simulink model "P7_Cascade_Control"  (R2023b)
settings: Solver=FixedStepAuto  StartTime=0.0  StopTime=20e-3  FixedStep=1e-8  RelTol=1e-3
values from neighbouring files (symbols this model uses):
  L = 2e-3    (= 0.002)    [P7_T1_Buck_Single_Loop.m]
libraries: spsSeriesRLCBranchLib x9, spsMeanLib x6, spsCurrentMeasurementLib x3, spsDiodeLib x3, spsIdealSwitchLib x3, eePwmGenerator x3, spsDCVoltageSourceLib x3, spsVoltageMeasurementLib x3, slpidlib x2, sps_lib x1
settings Model: Creator=Lucas  LastModifiedBy=Lucas
settings SolverCC: ZeroCrossAlgorithm=Adaptive
settings DebuggingCC: IgnoredZcDiagnostic=none

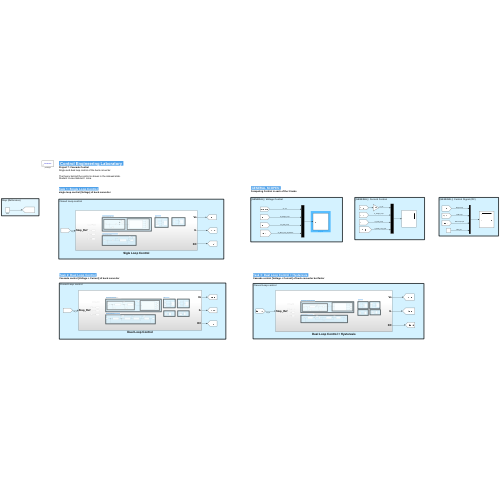
[thumbnail: Simulink's stored preview of the top-level diagram]
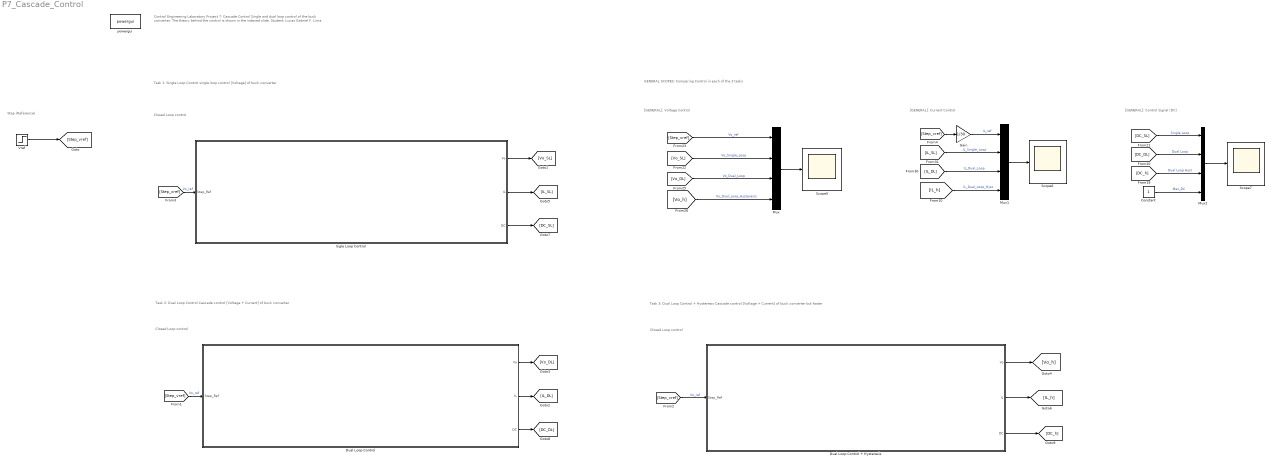
== system P7_Cascade_Control ==
  note: Control Engineering Laboratory
      | Project 7: Cascade Control
      | Single and dual loop control of the buck converter.
      |
      | The theory behind the control is shown in the indexed slide.
      | Student: Lucas Gabriel F. Lima.
  note: Step (Reference)
  note: [GENERAL]: Voltage Control
  note: [GENERAL]: Current Control
  note: [GENERAL]: Control Signal (DC)
  note: GENERAL SCOPES:
      | Comparing Control in each of the 3 tasks
  note: Task 2: Dual Loop Control
      | Cascade control [Voltage + Current] of buck converter
  note: Task 3: Dual Loop Control + Hysteresis
      | Cascade control [Voltage + Current] of buck converter but faster
  note: Task 1: Single Loop Control
      | single loop control [Voltage] of buck converter
  note: Closed Loop control
  note: Closed Loop control
  note: Closed Loop control
  Constant : Constant
  Dual Loop Control : Subsystem
  Dual Loop Control + Hysteresis : Subsystem
  Gain : Gain  Gain=1/30
  Mux : Mux
  Mux1 : Mux
  Mux2 : Mux
  Scope5 : Scope
  Scope6 : Scope
  Scope7 : Scope
  Sigle Loop Control : Subsystem
  Vref : Step  Time=10e-3  Before=60  After=66  SampleTime=0
  powergui : sps_lib/powergui  Priority=1  SimulationMode=Continuous  SampleTime=50e-6  frequency=60  Iterations=50  frequencyindice=0  Pbase=100e6  ErrMax=1e-4  UnitsV=kV  UnitsW=MW  buscounter=0  FunctionMessages=off  echomessages=off  EnableUseOfTLC=off  CurrentSourceSwitches=off  DisableSnubberDevices=off  DisableRonSwitches=off  DisableVfSwitches=off  DisplayEquations=off  AutomaticDiscreteSolvers=off  SolverType=Tustin/Backward Euler (TBE)  Interpol=off  ExternalGateDelay=off  methode=off  Ts=100  x0status=blocks  SPID=on  SwTol=0  HookPort=off  NonlinearTolerance=1e-4  nMaxIteration=100  ContinueOnMaxIteration=off  RestoreLinks=warning  ResistiveCurrentMeasurement=off  Frange=[0:2:500]  Ylog=off  Xlog=on  ShowGrid=off  save=off  variable=ZData  structure=0  ZoomFFT=off  StartTime=0.0  cycles=1  DisplayStyle=1  fundamental=60  FreqAxis=off  MaxFrequency=1000  frequencyindicesteady=1  RmsSteady=1  display=off
  wires:
  Vref/1 -> [Step_vref]
  [DC_h] -> Mux2/3  "Dual Loop Hyst"
  [DC_DL] -> Mux2/2  "Dual Loop"
  [DC_SL] -> Mux2/1  "Single Loop"
  [Vo_SL] -> Mux/2  "Vo_Single_Loop"
  [Step_vref] -> Mux/1  "Vo_ref"
  [Vo_DL] -> Mux/3  "Vo_Dual_Loop"
  [Vo_h] -> Mux/4  "Vo_Dual_Loop_Hysteresis"
  Mux/1 -> Scope5/1
  [IL_h] -> Mux1/4  "IL_Dual_Loop_Hyst"
  [IL_DL] -> Mux1/3  "IL_Dual_Loop"
  [IL_SL] -> Mux1/2  "IL_Single_Loop"
  Mux1/1 -> Scope6/1
  Mux2/1 -> Scope7/1
  Constant/1 -> Mux2/4  "Max_DC"
  [Step_vref] -> Dual Loop Control/1(Step_Ref)  "Vo_ref"
  Dual Loop Control/1(Vo) -> [Vo_DL]
  Dual Loop Control/2(IL) -> [IL_DL]
  [Step_vref] -> Dual Loop Control + Hysteresis/1(Step_Ref)  "Vo_ref"
  Dual Loop Control + Hysteresis/1(Vo) -> [Vo_h]
  Dual Loop Control + Hysteresis/2(IL) -> [IL_h]
  [Step_vref] -> Sigle Loop Control/1(Step_Ref)  "Vo_ref"
  Sigle Loop Control/1(Vo) -> [Vo_SL]
  Sigle Loop Control/2(IL) -> [IL_SL]
  Sigle Loop Control/3(DC) -> [DC_SL]
  Dual Loop Control/3(DC) -> [DC_DL]
  Dual Loop Control + Hysteresis/3(DC) -> [DC_h]
  [Step_vref] -> Gain/1
  Gain/1 -> Mux1/1  "IL_ref"

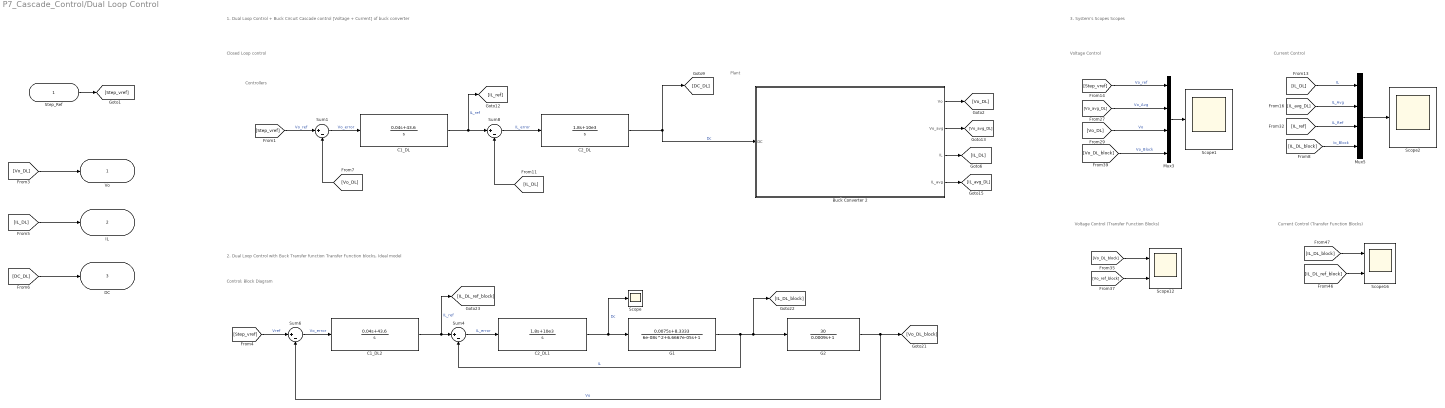
== system P7_Cascade_Control/Dual Loop Control ==
  note: Closed Loop control
  note: Control: Block Diagram
  note: Controllers
  note: Plant
  note: Voltage Control
  note: Current Control
  note: 1. Dual Loop Control + Buck Circuit
      | Cascade control [Voltage + Current] of buck converter
  note: 2. Dual Loop Control with Buck Transfer function
      | Transfer Function blocks, Ideal model
  note: 3. System's Scopes
      | Scopes
  note: Voltage Control (Transfer Function Blocks)
  note: Current Control (Transfer Function Blocks)
  Step_Ref : Inport
  Buck Converter 2 : Subsystem
  C1_DL : TransferFcn  Numerator=[0.04, 43.6]  Denominator=[1 , 0]
  C1_DL2 : TransferFcn  Numerator=[0.04, 43.6]  Denominator=[1 , 0]
  C2_DL : TransferFcn  Numerator=[1.8, 10e3]  Denominator=[1, 0]
  C2_DL1 : TransferFcn  Numerator=[1.8, 10e3]  Denominator=[1, 0]
  G1 : TransferFcn  Numerator=[0.0075, 8.3333]  Denominator=[6e-08, 6.6667e-05 ,1]
  G2 : TransferFcn  Numerator=30  Denominator=[0.0009 1]
  Mux3 : Mux
  Mux5 : Mux
  Scope : Scope
  Scope1 : Scope
  Scope12 : Scope  NumInputPorts=2
  Scope16 : Scope  NumInputPorts=2
  Scope2 : Scope
  Sum{1,4,6,8} (4 alike) : Sum  Inputs=|+-
  Vo : Outport
  IL : Outport  Port=2
  DC : Outport  Port=3
  wires:
  Sum6/1 -> C1_DL2/1  "Vo_error"
  Buck Converter 2/1(Vo) -> [Vo_DL]
  [IL_avg_DL] -> Mux5/2  "IL_Avg"
  [Step_vref] -> Sum6/1  "Vref"
  [Vo_DL] -> Sum1/2
  Sum4/1 -> C2_DL1/1  "IL_error"
  G1/1 -> [IL_DL_block], G2/1, Sum4/2  "IL"
  C1_DL2/1 -> [IL_DL_ref_block], Sum4/1  "IL_ref"
  [IL_DL] -> Mux5/1  "IL"
  [Vo_DL_block] -> Scope12/1
  Mux3/1 -> Scope1/1
  Sum1/1 -> C1_DL/1  "Vo_error"
  [IL_DL] -> Sum8/2
  Sum8/1 -> C2_DL/1  "IL_error"
  Buck Converter 2/3(IL) -> [IL_DL]
  C2_DL/1 -> Buck Converter 2/1(DC), [DC_DL]  "Dc"
  G2/1 -> [Vo_DL_block], Sum6/2  "Vo"
  C2_DL1/1 -> Scope/1, G1/1  "Dc"
  [IL_ref] -> Mux5/3  "IL_Ref"
  [Vo_ref_block] -> Scope12/2
  [Vo_avg_DL] -> Mux3/2  "Vo_Avg"
  Buck Converter 2/4(IL_avg) -> [IL_avg_DL]
  C1_DL/1 -> [IL_ref], Sum8/1  "IL_ref"
  [IL_DL_block] -> Scope16/1
  [Vo_DL] -> Mux3/3  "Vo"
  [Step_vref] -> Sum1/1  "Vo_ref"
  [Step_vref] -> Mux3/1  "Vo_ref"
  [Vo_DL_block] -> Mux3/4  "Vo_Block"
  Buck Converter 2/2(Vo_avg) -> [Vo_avg_DL]
  [IL_DL_block] -> Mux5/4  "Io_Block"
  Mux5/1 -> Scope2/1
  [IL_DL_ref_block] -> Scope16/2
  Step_Ref/1 -> [Step_vref]
  [Vo_DL] -> Vo/1
  [DC_DL] -> DC/1
  [IL_DL] -> IL/1

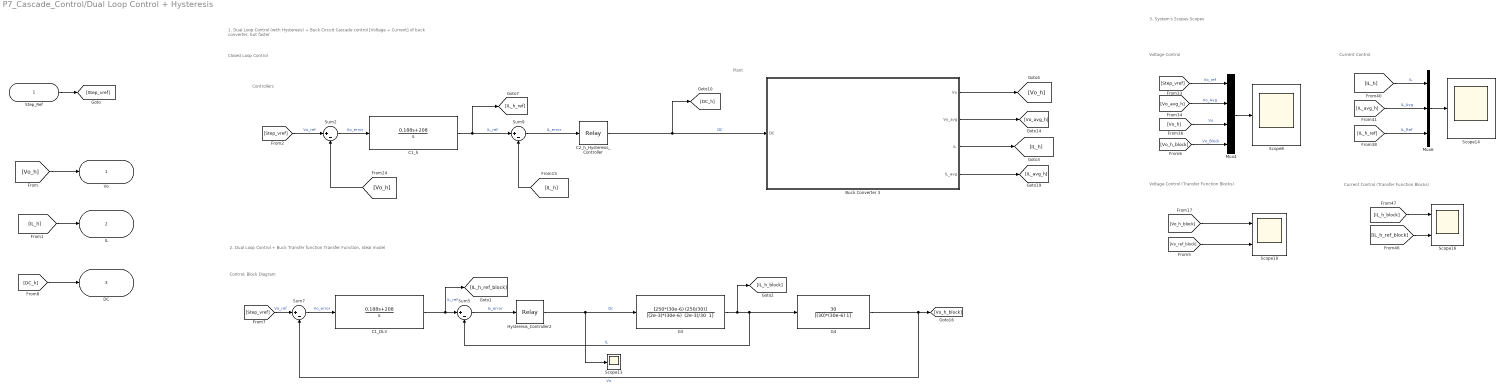
== system P7_Cascade_Control/Dual Loop Control + Hysteresis ==
  note: 2. Dual Loop Control + Buck Transfer function
      | Transfer Function, Ideal model
  note: Control: Block Diagram
  note: Controllers
  note: 1. Dual Loop Control (with Hysteresis) + Buck Circuit
      | Cascade control [Voltage + Current] of buck converter, but faster
  note: Voltage Control
  note: Plant
  note: Current Control
  note: Closed Loop Control
  note: 3. System's Scopes
      | Scopes
  note: Voltage Control (Transfer Function Blocks)
  note: Current Control (Transfer Function Blocks)
  Step_Ref : Inport
  Buck Converter 3 : Subsystem
  C1_DL3 : TransferFcn  Numerator=[0.188 , 208]  Denominator=[1 , 0]
  C1_h : TransferFcn  Numerator=[0.188 , 208]  Denominator=[1 , 0]
  C2_h_Hysteresis_Controller : Relay  OnSwitchValue=0.2/2  OffSwitchValue=-0.2/2
  G3 : TransferFcn  Numerator=[250*(30e-6) (250/30)]  Denominator="[(2e-3)*(30e-6)  (2e-3)/30  1]"
  G4 : TransferFcn  Numerator=30  Denominator=[(30)*(30e-6) 1]
  Hysteresis_Controller2 : Relay  OnSwitchValue=0.2/2  OffSwitchValue=-0.2/2
  Mux4 : Mux
  Mux6 : Mux  Inputs=3
  Scope10 : Scope  NumInputPorts=2
  Scope13 : Scope
  Scope14 : Scope
  Scope16 : Scope  NumInputPorts=2
  Scope8 : Scope
  Sum{2,5,7,9} (4 alike) : Sum  Inputs=|+-
  Vo : Outport
  IL : Outport  Port=2
  DC : Outport  Port=3
  wires:
  G3/1 -> [IL_h_block], G4/1, Sum5/2  "IL"
  Sum7/1 -> C1_DL3/1  "Vo_error"
  C1_DL3/1 -> [IL_h_ref_block], Sum5/1  "IL_ref"
  C1_h/1 -> [IL_h_ref], Sum9/1  "IL_ref"
  G4/1 -> Sum7/2, [Vo_h_block]  "Vo"
  [Vo_ref_block] -> Scope10/2
  [Vo_avg_h] -> Mux4/2  "Vo_Avg"
  [Vo_h_block] -> Scope10/1
  Buck Converter 3/3(IL) -> [IL_h]
  Mux4/1 -> Scope8/1
  Sum5/1 -> Hysteresis_Controller2/1  "Io_error"
  [IL_h] -> Sum9/2
  C2_h_Hysteresis_Controller/1 -> Buck Converter 3/1(DC), [DC_h]  "DC"
  Buck Converter 3/1(Vo) -> [Vo_h]
  [Vo_h] -> Sum2/2
  [Vo_h] -> Mux4/3  "Vo"
  Sum9/1 -> C2_h_Hysteresis_Controller/1  "IL_error"
  [IL_avg_h] -> Mux6/2  "IL_Avg"
  Sum2/1 -> C1_h/1  "Vo_error"
  [IL_h_ref] -> Mux6/3  "IL_Ref"
  Buck Converter 3/4(IL_avg) -> [IL_avg_h]
  Mux6/1 -> Scope14/1
  Buck Converter 3/2(Vo_avg) -> [Vo_avg_h]
  [Step_vref] -> Mux4/1  "Vo_ref"
  Hysteresis_Controller2/1 -> Scope13/1, G3/1  "Dc"
  [Step_vref] -> Sum2/1  "Vo_ref"
  [IL_h] -> Mux6/1  "IL"
  Step_Ref/1 -> [Step_vref]
  [Vo_h] -> Vo/1
  [Vo_h_block] -> Mux4/4  "Vo_Block"
  [Step_vref] -> Sum7/1  "Vo_ref"
  [DC_h] -> DC/1
  [IL_h_ref_block] -> Scope16/2
  [IL_h_block] -> Scope16/1
  [IL_h] -> IL/1

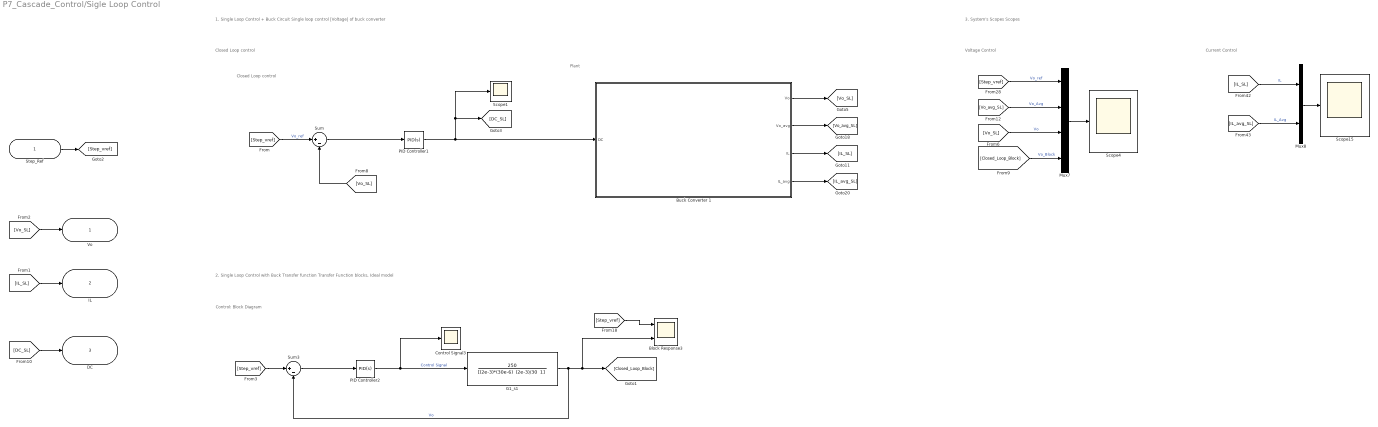
== system P7_Cascade_Control/Sigle Loop Control ==
  note: Closed Loop control
  note: Control: Block Diagram
  note: Voltage Control
  note: Current Control
  note: Plant
  note: Closed Loop control
  note: 1. Single Loop Control + Buck Circuit
      | Single loop control [Voltage] of buck converter
  note: 2. Single Loop Control with Buck Transfer function
      | Transfer Function blocks, Ideal model
  note: 3. System's Scopes
      | Scopes
  Step_Ref : Inport
  Block Response3 : Scope  NumInputPorts=2
  Buck Converter 1 : Subsystem
  Control Signal3 : Scope
  G1_s1 : TransferFcn  Numerator=250  Denominator="[(2e-3)*(30e-6)  (2e-3)/30  1]"
  Mux7 : Mux
  Mux8 : Mux  Inputs=2
  PID Controller1 : slpidlib/PID Controller  Controller=PID  Form=Parallel  TimeDomain=Continuous-time  UseExternalTs=off  SampleTime=-1  IntegratorMethod=Forward Euler  FilterMethod=Forward Euler  ControllerParametersSource=internal  P=0.0075  I=14  UseKiTs=off  D=0.8e-06  N=1/(8.18e-06)  UseFilter=on  TunerSelectOption=Transfer Function Based (PID Tuner App)  InitialConditionSource=internal  InitialConditionForIntegrator=0  InitialConditionForFilter=0  DifferentiatorICPrevScaledInput=0  ExternalReset=none  TrackingMode=off  Kt=1  LimitOutput=off  SatLimitsSource=internal  UpperSaturationLimit=inf  LowerSaturationLimit=-inf  LinearizeAsGain=on  AntiWindupMode=none  Kb=1  LimitIntegrator=off  UpperIntegratorSaturationLimit=inf  LowerIntegratorSaturationLimit=-inf  POutMin=[]  POutMax=[]  IOutMin=[]  IOutMax=[]  DOutMin=[]  DOutMax=[]  NOutMin=[]  NOutMax=[]  SumOutMin=[]  SumOutMax=[]  SaturationOutMin=[]  SaturationOutMax=[]  PParamMin=[]  PParamMax=[]  IParamMin=[]  IParamMax=[]  DParamMin=[]  DParamMax=[]  NParamMin=[]  NParamMax=[]  KbParamMin=[]  KbParamMax=[]  KtParamMin=[]  KtParamMax=[]  KbOutMin=[]  KbOutMax=[]  KtOutMin=[]  KtOutMax=[]  IntegratorOutMin=[]  IntegratorOutMax=[]  FilterOutMin=[]  FilterOutMax=[]  SumI1OutMin=[]  SumI1OutMax=[]  SumI2OutMin=[]  SumI2OutMax=[]  SumI3OutMin=[]  SumI3OutMax=[]  SumI4OutMin=[]  SumI4OutMax=[]  SumDOutMin=[]  SumDOutMax=[]  DifferentiatorOutMin=[]  DifferentiatorOutMax=[]  FilterDiffOutCoefMin=[]  FilterDiffOutCoefMax=[]  ReciprocalOutMin=[]  ReciprocalOutMax=[]  SumDenOutMin=[]  SumDenOutMax=[]  SumNumOutMin=[]  SumNumOutMax=[]  DivideOutMin=[]  DivideOutMax=[]  UdiffTsProdOutMin=[]  UdiffTsProdOutMax=[]  NTsProdOutMin=[]  NTsProdOutMax=[]  UintegralTsProdOutMin=[]  UintegralTsProdOutMax=[]  UngainTsProdOutMin=[]  UngainTsProdOutMax=[]  ClampingZeroOutDataTypeStr=Inherit: Inherit via back propagation  ClampingZeroOutMin=[]  ClampingZeroOutMax=[]  FilterDenConstantOutDataTypeStr=Inherit: Inherit via back propagation  FilterDenConstantOutMin=[]  FilterDenConstantOutMax=[]  PCopyOutDataTypeStr=Inherit: Inherit via back propagation  PCopyOutMin=[]  PCopyOutMax=[]  NCopyOutDataTypeStr=Inherit: Inherit via back propagation  NCopyOutMin=[]  NCopyOutMax=[]  IntegratorContinuousStateAttributes=''  IntegratorStateMustResolveToSignalObject=off  IntegratorRTWStateStorageClass=Auto  FilterContinuousStateAttributes=''  FilterStateMustResolveToSignalObject=off  FilterRTWStateStorageClass=Auto  ParallelPVariant=InternalParameters  IdealPVariant=Disabled  IVariant=InternalParameters  DVariant=InternalParameters  IntegratorVariant=Continuous  SatVariant=Disabled  AWVariant=Passthrough  PCopyVariant=Disabled  TRVariant=Disabled  FdbkBlocksVariant=Forward  IdealPFdbkVariant=Disabled  SatFdbkVariant=Disabled  DerivativeFilterVariant=ContFilter  NVariant=InternalParameters  NCopyVariant=Disabled  FilterICVariant=InternalICsFilter  IntegratorICVariant=InternalICs  ExternalResetVariant=Disabled  TRSumVariant=Passthrough  SumFdbkVariant=Disabled  SumVariant=Sum_PID  TsampFilterVariant=InternalTs  TsampNgainVariant=Passthrough  TsampIntegralVariant=Disabled_SignalSpec  ExternalSaturationOutDataTypeStr=Inherit: Same as second input
  PID Controller2 : slpidlib/PID Controller  Controller=PID  Form=Parallel  TimeDomain=Continuous-time  UseExternalTs=off  SampleTime=-1  IntegratorMethod=Forward Euler  FilterMethod=Forward Euler  ControllerParametersSource=internal  P=0.0075  I=14  UseKiTs=off  D=0.8e-06  N=1/(8.18e-06)  UseFilter=on  TunerSelectOption=Transfer Function Based (PID Tuner App)  InitialConditionSource=internal  InitialConditionForIntegrator=0  InitialConditionForFilter=0  DifferentiatorICPrevScaledInput=0  ExternalReset=none  TrackingMode=off  Kt=1  LimitOutput=off  SatLimitsSource=internal  UpperSaturationLimit=inf  LowerSaturationLimit=-inf  LinearizeAsGain=on  AntiWindupMode=none  Kb=1  LimitIntegrator=off  UpperIntegratorSaturationLimit=inf  LowerIntegratorSaturationLimit=-inf  POutMin=[]  POutMax=[]  IOutMin=[]  IOutMax=[]  DOutMin=[]  DOutMax=[]  NOutMin=[]  NOutMax=[]  SumOutMin=[]  SumOutMax=[]  SaturationOutMin=[]  SaturationOutMax=[]  PParamMin=[]  PParamMax=[]  IParamMin=[]  IParamMax=[]  DParamMin=[]  DParamMax=[]  NParamMin=[]  NParamMax=[]  KbParamMin=[]  KbParamMax=[]  KtParamMin=[]  KtParamMax=[]  KbOutMin=[]  KbOutMax=[]  KtOutMin=[]  KtOutMax=[]  IntegratorOutMin=[]  IntegratorOutMax=[]  FilterOutMin=[]  FilterOutMax=[]  SumI1OutMin=[]  SumI1OutMax=[]  SumI2OutMin=[]  SumI2OutMax=[]  SumI3OutMin=[]  SumI3OutMax=[]  SumI4OutMin=[]  SumI4OutMax=[]  SumDOutMin=[]  SumDOutMax=[]  DifferentiatorOutMin=[]  DifferentiatorOutMax=[]  FilterDiffOutCoefMin=[]  FilterDiffOutCoefMax=[]  ReciprocalOutMin=[]  ReciprocalOutMax=[]  SumDenOutMin=[]  SumDenOutMax=[]  SumNumOutMin=[]  SumNumOutMax=[]  DivideOutMin=[]  DivideOutMax=[]  UdiffTsProdOutMin=[]  UdiffTsProdOutMax=[]  NTsProdOutMin=[]  NTsProdOutMax=[]  UintegralTsProdOutMin=[]  UintegralTsProdOutMax=[]  UngainTsProdOutMin=[]  UngainTsProdOutMax=[]  ClampingZeroOutDataTypeStr=Inherit: Inherit via back propagation  ClampingZeroOutMin=[]  ClampingZeroOutMax=[]  FilterDenConstantOutDataTypeStr=Inherit: Inherit via back propagation  FilterDenConstantOutMin=[]  FilterDenConstantOutMax=[]  PCopyOutDataTypeStr=Inherit: Inherit via back propagation  PCopyOutMin=[]  PCopyOutMax=[]  NCopyOutDataTypeStr=Inherit: Inherit via back propagation  NCopyOutMin=[]  NCopyOutMax=[]  IntegratorContinuousStateAttributes=''  IntegratorStateMustResolveToSignalObject=off  IntegratorRTWStateStorageClass=Auto  FilterContinuousStateAttributes=''  FilterStateMustResolveToSignalObject=off  FilterRTWStateStorageClass=Auto  ParallelPVariant=InternalParameters  IdealPVariant=Disabled  IVariant=InternalParameters  DVariant=InternalParameters  IntegratorVariant=Continuous  SatVariant=Disabled  AWVariant=Passthrough  PCopyVariant=Disabled  TRVariant=Disabled  FdbkBlocksVariant=Forward  IdealPFdbkVariant=Disabled  SatFdbkVariant=Disabled  DerivativeFilterVariant=ContFilter  NVariant=InternalParameters  NCopyVariant=Disabled  FilterICVariant=InternalICsFilter  IntegratorICVariant=InternalICs  ExternalResetVariant=Disabled  TRSumVariant=Passthrough  SumFdbkVariant=Disabled  SumVariant=Sum_PID  TsampFilterVariant=InternalTs  TsampNgainVariant=Passthrough  TsampIntegralVariant=Disabled_SignalSpec  ExternalSaturationOutDataTypeStr=Inherit: Same as second input
  Scope1 : Scope
  Scope15 : Scope
  Scope4 : Scope
  Sum : Sum  Inputs=|+-
  Sum3 : Sum  Inputs=|+-
  Vo : Outport
  IL : Outport  Port=2
  DC : Outport  Port=3
  wires:
  G1_s1/1 -> [Closed_Loop_Block], Block Response3/2, Sum3/2  "Vo"
  Sum/1 -> PID Controller1/1
  Mux7/1 -> Scope4/1
  Buck Converter 1/1(Vo) -> [Vo_SL]
  [Step_vref] -> Sum/1  "Vo_ref"
  [Vo_SL] -> Sum/2
  [Step_vref] -> Sum3/1
  [Vo_SL] -> Mux7/3  "Vo"
  [IL_SL] -> Mux8/1  "IL"
  [IL_avg_SL] -> Mux8/2  "IL_Avg"
  [Step_vref] -> Block Response3/1
  Buck Converter 1/2(Vo_avg) -> [Vo_avg_SL]
  [Step_vref] -> Mux7/1  "Vo_ref"
  [Closed_Loop_Block] -> Mux7/4  "Vo_Block"
  [Vo_avg_SL] -> Mux7/2  "Vo_Avg"
  Buck Converter 1/3(IL) -> [IL_SL]
  Buck Converter 1/4(IL_avg) -> [IL_avg_SL]
  Mux8/1 -> Scope15/1
  PID Controller2/1 -> G1_s1/1, Control Signal3/1  "Control Signal"
  Sum3/1 -> PID Controller2/1
  Step_Ref/1 -> [Step_vref]
  [DC_SL] -> DC/1
  PID Controller1/1 -> Buck Converter 1/1(DC), Scope1/1, [DC_SL]
  [IL_SL] -> IL/1
  [Vo_SL] -> Vo/1

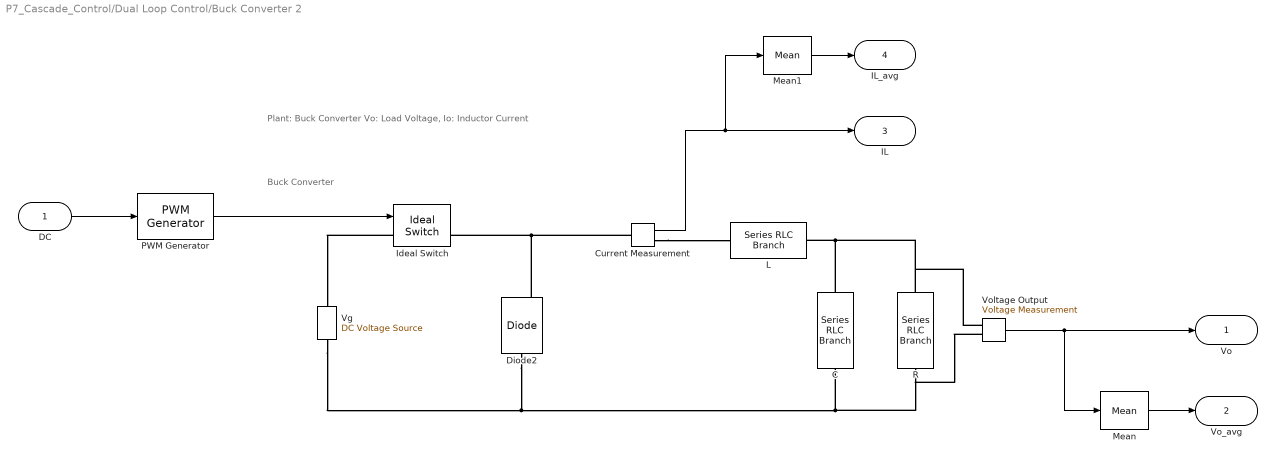
== system P7_Cascade_Control/Dual Loop Control/Buck Converter 2 ==
  note: Plant: Buck Converter
      | Vo: Load Voltage, Io: Inductor Current
  note: Buck Converter
  DC : Inport
  C : spsSeriesRLCBranchLib/Series RLC Branch  LConnTagsString=__new0  RConnTagsString=__new0  BranchType=C  Resistance=1  Inductance=L  SetiL0=off  InitialCurrent=0  Capacitance=30e-6  Setx0=off  InitialVoltage=0  Measurements=None
  Current Measurement : spsCurrentMeasurementLib/Current Measurement  PhasorSimulation=off  OutputType=Complex  PSBequivalent=0
  Diode2 : spsDiodeLib/Diode  Ron=0.00001  Lon=0  Vf=0  IC=0  UseSnubber=0  Rs=inf  Cs=inf  Measurements=on
  Ideal Switch : spsIdealSwitchLib/Ideal Switch  Ron=0.001  Lon=0  IC=0  Rs=1e5  Cs=inf  Measurements=on
  L : spsSeriesRLCBranchLib/Series RLC Branch  LConnTagsString=__new0  RConnTagsString=__new0  BranchType=L  Resistance=1  Inductance=2e-3  SetiL0=off  InitialCurrent=0  Capacitance=1e-6  Setx0=off  InitialVoltage=0  Measurements=None
  Mean : spsMeanLib/Mean  Freq=(10e3)  Vinit=0  Ts=0
  Mean1 : spsMeanLib/Mean  Freq=(10e3)  Vinit=0  Ts=0
  PWM Generator : eePwmGenerator/PWM Generator  CarrCount=Up  Tper=1/(10e3)  Tdelay=0  Ts=0
  R : spsSeriesRLCBranchLib/Series RLC Branch  LConnTagsString=__new0  RConnTagsString=__new0  BranchType=R  Resistance=30  Inductance=L  SetiL0=off  InitialCurrent=0  Capacitance=1e-6  Setx0=off  InitialVoltage=0  Measurements=None
  Vg : spsDCVoltageSourceLib/DC Voltage Source  Amplitude=250  Measurements=None
  Voltage Output : spsVoltageMeasurementLib/Voltage Measurement  PhasorSimulation=off  OutputType=Complex  PSBequivalent=0
  Vo : Outport
  Vo_avg : Outport  Port=2
  IL : Outport  Port=3
  IL_avg : Outport  Port=4
  wires:
  Voltage Output/1 -> Vo/1, Mean/1
  Mean/1 -> Vo_avg/1
  Current Measurement/1 -> IL/1, Mean1/1
  DC/1 -> PWM Generator/1
  PWM Generator/1 -> Ideal Switch/1
  Mean1/1 -> IL_avg/1
  connections:
  Vg/LConn1 -- Diode2/LConn1 -- C/RConn1 -- R/RConn1 -- Voltage Output/LConn2
  Current Measurement/LConn1 -- Ideal Switch/RConn1 -- Diode2/RConn1
  C/LConn1 -- L/RConn1 -- R/LConn1 -- Voltage Output/LConn1
  Ideal Switch/LConn1 -- Vg/RConn1
  Current Measurement/RConn1 -- L/LConn1

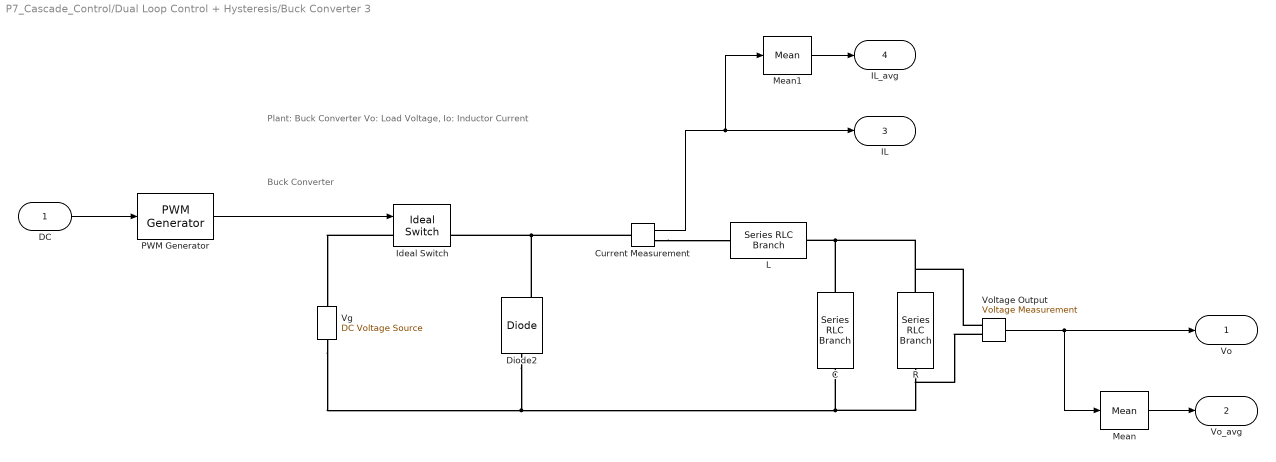
== system P7_Cascade_Control/Dual Loop Control + Hysteresis/Buck Converter 3 ==
  note: Plant: Buck Converter
      | Vo: Load Voltage, Io: Inductor Current
  note: Buck Converter
  DC : Inport
  C : spsSeriesRLCBranchLib/Series RLC Branch  LConnTagsString=__new0  RConnTagsString=__new0  BranchType=C  Resistance=1  Inductance=L  SetiL0=off  InitialCurrent=0  Capacitance=30e-6  Setx0=off  InitialVoltage=0  Measurements=None
  Current Measurement : spsCurrentMeasurementLib/Current Measurement  PhasorSimulation=off  OutputType=Complex  PSBequivalent=0
  Diode2 : spsDiodeLib/Diode  Ron=0.00001  Lon=0  Vf=0  IC=0  UseSnubber=0  Rs=inf  Cs=inf  Measurements=on
  Ideal Switch : spsIdealSwitchLib/Ideal Switch  Ron=0.001  Lon=0  IC=0  Rs=1e5  Cs=inf  Measurements=on
  L : spsSeriesRLCBranchLib/Series RLC Branch  LConnTagsString=__new0  RConnTagsString=__new0  BranchType=L  Resistance=1  Inductance=2e-3  SetiL0=off  InitialCurrent=0  Capacitance=1e-6  Setx0=off  InitialVoltage=0  Measurements=None
  Mean : spsMeanLib/Mean  Freq=(10e3)  Vinit=0  Ts=0
  Mean1 : spsMeanLib/Mean  Freq=(10e3)  Vinit=0  Ts=0
  PWM Generator : eePwmGenerator/PWM Generator  CarrCount=Up  Tper=1/(10e3)  Tdelay=0  Ts=0
  R : spsSeriesRLCBranchLib/Series RLC Branch  LConnTagsString=__new0  RConnTagsString=__new0  BranchType=R  Resistance=30  Inductance=L  SetiL0=off  InitialCurrent=0  Capacitance=1e-6  Setx0=off  InitialVoltage=0  Measurements=None
  Vg : spsDCVoltageSourceLib/DC Voltage Source  Amplitude=250  Measurements=None
  Voltage Output : spsVoltageMeasurementLib/Voltage Measurement  PhasorSimulation=off  OutputType=Complex  PSBequivalent=0
  Vo : Outport
  Vo_avg : Outport  Port=2
  IL : Outport  Port=3
  IL_avg : Outport  Port=4
  wires:
  Voltage Output/1 -> Vo/1, Mean/1
  Mean/1 -> Vo_avg/1
  Current Measurement/1 -> IL/1, Mean1/1
  DC/1 -> PWM Generator/1
  PWM Generator/1 -> Ideal Switch/1
  Mean1/1 -> IL_avg/1
  connections:
  Vg/LConn1 -- Diode2/LConn1 -- C/RConn1 -- R/RConn1 -- Voltage Output/LConn2
  Current Measurement/LConn1 -- Ideal Switch/RConn1 -- Diode2/RConn1
  C/LConn1 -- L/RConn1 -- R/LConn1 -- Voltage Output/LConn1
  Ideal Switch/LConn1 -- Vg/RConn1
  Current Measurement/RConn1 -- L/LConn1

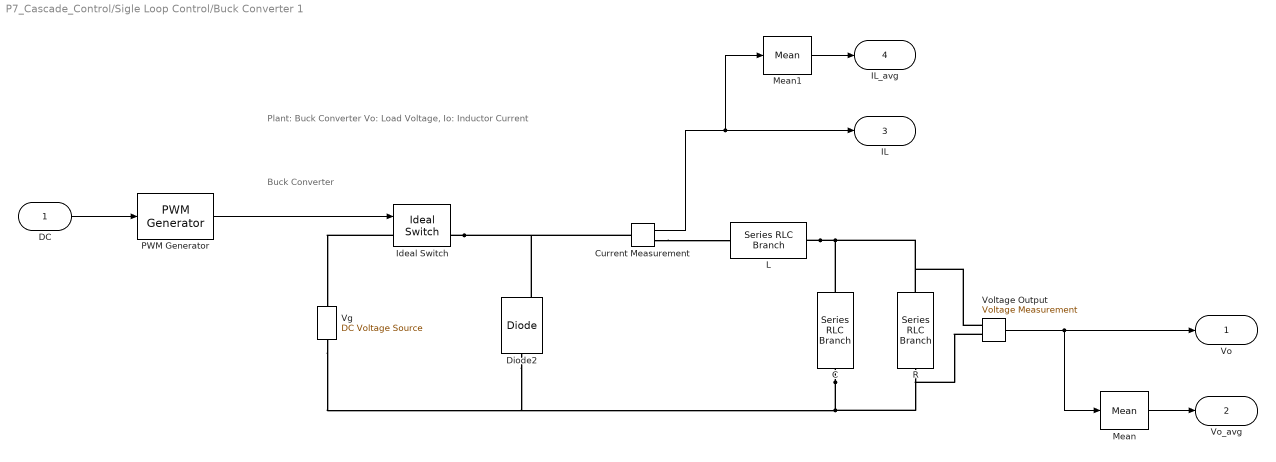
== system P7_Cascade_Control/Sigle Loop Control/Buck Converter 1 ==
  note: Plant: Buck Converter
      | Vo: Load Voltage, Io: Inductor Current
  note: Buck Converter
  DC : Inport
  C : spsSeriesRLCBranchLib/Series RLC Branch  LConnTagsString=__new0  RConnTagsString=__new0  BranchType=C  Resistance=1  Inductance=L  SetiL0=off  InitialCurrent=0  Capacitance=30e-6  Setx0=off  InitialVoltage=0  Measurements=None
  Current Measurement : spsCurrentMeasurementLib/Current Measurement  PhasorSimulation=off  OutputType=Complex  PSBequivalent=0
  Diode2 : spsDiodeLib/Diode  Ron=0.00001  Lon=0  Vf=0  IC=0  UseSnubber=0  Rs=inf  Cs=inf  Measurements=on
  Ideal Switch : spsIdealSwitchLib/Ideal Switch  Ron=0.001  Lon=0  IC=0  Rs=1e5  Cs=inf  Measurements=on
  L : spsSeriesRLCBranchLib/Series RLC Branch  LConnTagsString=__new0  RConnTagsString=__new0  BranchType=L  Resistance=1  Inductance=2e-3  SetiL0=off  InitialCurrent=0  Capacitance=1e-6  Setx0=off  InitialVoltage=0  Measurements=None
  Mean : spsMeanLib/Mean  Freq=(10e3)  Vinit=0  Ts=0
  Mean1 : spsMeanLib/Mean  Freq=(10e3)  Vinit=0  Ts=0
  PWM Generator : eePwmGenerator/PWM Generator  CarrCount=Up  Tper=1/(10e3)  Tdelay=0  Ts=0
  R : spsSeriesRLCBranchLib/Series RLC Branch  LConnTagsString=__new0  RConnTagsString=__new0  BranchType=R  Resistance=30  Inductance=L  SetiL0=off  InitialCurrent=0  Capacitance=1e-6  Setx0=off  InitialVoltage=0  Measurements=None
  Vg : spsDCVoltageSourceLib/DC Voltage Source  Amplitude=250  Measurements=None
  Voltage Output : spsVoltageMeasurementLib/Voltage Measurement  PhasorSimulation=off  OutputType=Complex  PSBequivalent=0
  Vo : Outport
  Vo_avg : Outport  Port=2
  IL : Outport  Port=3
  IL_avg : Outport  Port=4
  wires:
  Voltage Output/1 -> Vo/1, Mean/1
  Mean/1 -> Vo_avg/1
  Current Measurement/1 -> IL/1, Mean1/1
  DC/1 -> PWM Generator/1
  PWM Generator/1 -> Ideal Switch/1
  Mean1/1 -> IL_avg/1
  connections:
  C/RConn1 -- R/RConn1 -- Voltage Output/LConn2 -- Vg/LConn1 -- Diode2/LConn1
  Ideal Switch/RConn1 -- Current Measurement/LConn1 -- Diode2/RConn1
  L/RConn1 -- R/LConn1 -- Voltage Output/LConn1 -- C/LConn1
  Ideal Switch/LConn1 -- Vg/RConn1
  Current Measurement/RConn1 -- L/LConn1
